simulink model "calcul_alpha_beta_gamma_v2"  (R2024b)
settings: Solver=FixedStepDiscrete  StartTime=0.0  StopTime=10.0  FixedStep=Ts  RelTol=1e-3
values from neighbouring files (symbols this model uses):
  lf = L*fr    (= 0.7905)    [main_data_vehicle.m]    (also in xopt_launch.mat)
  lr = L-lf    (= 0.7595)    [main_data_vehicle.m]    (also in xopt_launch.mat)
settings Model: Creator=marti  LastModifiedBy=marti

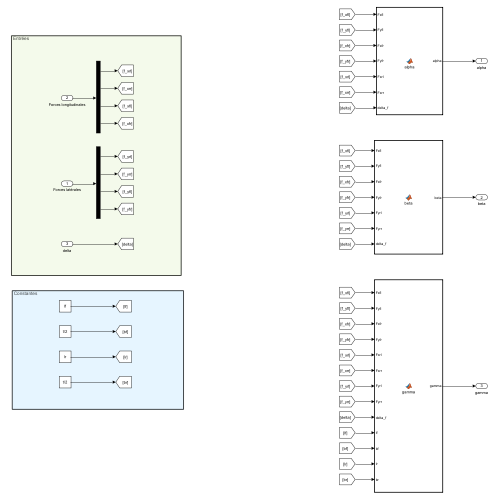
[thumbnail: Simulink's stored preview of the top-level diagram]
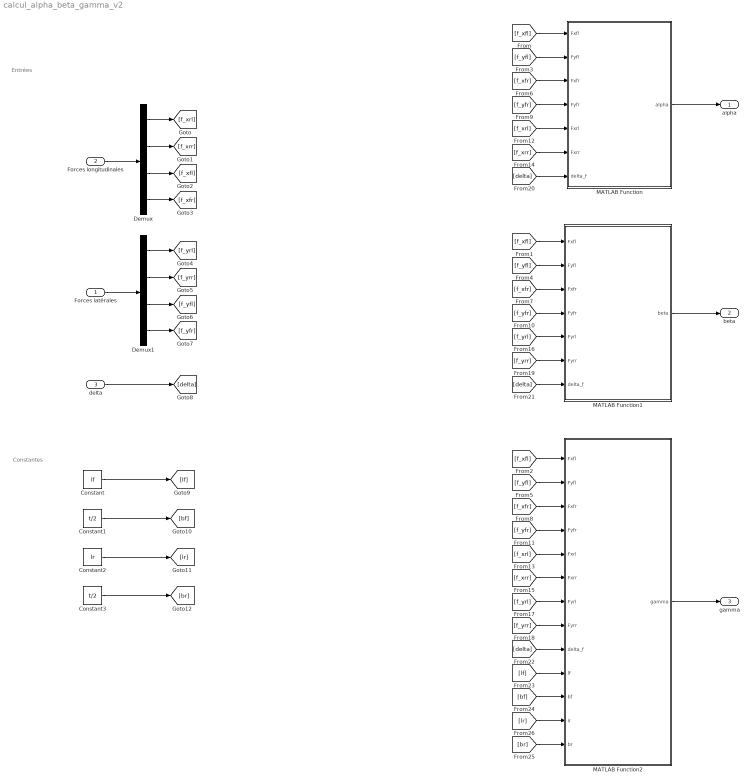
== system calcul_alpha_beta_gamma_v2 ==
  note: Constantes
  note: Entrées
  Forces latérales : Inport
  Forces longitudinales : Inport  Port=2
  delta : Inport  Port=3
  Constant : Constant  Value=lf
  Constant1 : Constant  Value=t/2
  Constant2 : Constant  Value=lr
  Constant3 : Constant  Value=t/2
  Demux : Demux
  Demux1 : Demux
  MATLAB Function : MATLAB Function  TreatAsAtomicUnit=on
  MATLAB Function1 : MATLAB Function  TreatAsAtomicUnit=on
  MATLAB Function2 : MATLAB Function  TreatAsAtomicUnit=on
  alpha : Outport
  beta : Outport  Port=2
  gamma : Outport  Port=3
  wires:
  Forces longitudinales/1 -> Demux/1
  Demux/1 -> [f_xrl]
  Demux/2 -> [f_xrr]
  Demux/3 -> [f_xfl]
  Demux/4 -> [f_xfr]
  Demux1/3 -> [f_yfl]
  Demux1/4 -> [f_yfr]
  Demux1/1 -> [f_yrl]
  Forces latérales/1 -> Demux1/1
  Demux1/2 -> [f_yrr]
  Constant/1 -> [lf]
  Constant1/1 -> [bf]
  Constant2/1 -> [lr]
  Constant3/1 -> [br]
  [f_xfl] -> MATLAB Function/1(Fxfl)
  [f_xfl] -> MATLAB Function1/1(Fxfl)
  [f_xfl] -> MATLAB Function2/1(Fxfl)
  [f_yfl] -> MATLAB Function/2(Fyfl)
  [f_yfl] -> MATLAB Function1/2(Fyfl)
  [f_yfl] -> MATLAB Function2/2(Fyfl)
  [f_xfr] -> MATLAB Function/3(Fxfr)
  [f_xfr] -> MATLAB Function1/3(Fxfr)
  [f_xfr] -> MATLAB Function2/3(Fxfr)
  [f_yfr] -> MATLAB Function/4(Fyfr)
  [f_yfr] -> MATLAB Function1/4(Fyfr)
  [f_yfr] -> MATLAB Function2/4(Fyfr)
  [f_xrl] -> MATLAB Function/5(Fxrl)
  [f_xrl] -> MATLAB Function2/5(Fxrl)
  [f_xrr] -> MATLAB Function/6(Fxrr)
  [f_xrr] -> MATLAB Function2/6(Fxrr)
  [f_yrl] -> MATLAB Function1/5(Fyrl)
  [f_yrl] -> MATLAB Function2/7(Fyrl)
  [f_yrr] -> MATLAB Function2/8(Fyrr)
  [f_yrr] -> MATLAB Function1/6(Fyrr)
  [delta] -> MATLAB Function/7(delta_f)
  [delta] -> MATLAB Function1/7(delta_f)
  [delta] -> MATLAB Function2/9(delta_f)
  [lf] -> MATLAB Function2/10(lf)
  [bf] -> MATLAB Function2/11(bf)
  [br] -> MATLAB Function2/13(br)
  [lr] -> MATLAB Function2/12(lr)
  MATLAB Function/1(alpha) -> alpha/1
  MATLAB Function1/1(beta) -> beta/1
  MATLAB Function2/1(gamma) -> gamma/1
  delta/1 -> [delta]

== matlab function calcul_alpha_beta_gamma_v2/MATLAB Function1 ==
  data: Fxfl input; beta output; Fyfl input; Fxfr input; Fyfr input; Fyrl input; Fyrr input; delta_f input
function beta = beta(Fxfl, Fyfl, Fxfr, Fyfr, Fyrl, Fyrr, delta_f)
% Calcule le terme de droite de la deuxième équation du système
% beta = Fxfl*sin(delta_f) + Fyfl*cos(delta_f) + Fxfr*sin(delta_f) + Fyfr*cos(delta_f) + Fyrl + Fyrr

beta = Fxfl*sin(delta_f) + Fyfl*cos(delta_f) + ...
       Fxfr*sin(delta_f) + Fyfr*cos(delta_f) + ...
       Fyrl + Fyrr;
end

== matlab function calcul_alpha_beta_gamma_v2/MATLAB Function ==
  data: Fxfl input; alpha output; Fyfl input; Fxfr input; Fyfr input; Fxrl input; Fxrr input; delta_f input
function alpha = alpha(Fxfl, Fyfl, Fxfr, Fyfr, Fxrl, Fxrr, delta_f)
% Calcule le terme de droite de la première équation du système
% alpha = Fxfl*cos(delta_f) - Fyfl*sin(delta_f) + Fxfr*cos(delta_f) - Fyfr*sin(delta_f) + Fxrl + Fxrr

alpha = Fxfl*cos(delta_f) - Fyfl*sin(delta_f) + ...
        Fxfr*cos(delta_f) - Fyfr*sin(delta_f) + ...
        Fxrl + Fxrr;
end

== matlab function calcul_alpha_beta_gamma_v2/MATLAB Function2 ==
  data: Fxfl input; gamma output; Fyfl input; Fxfr input; Fyfr input; Fxrl input; Fxrr input; Fyrl input; Fyrr input; delta_f input; lf input; bf input; lr input; br input
function gamma = gamma(Fxfl, Fyfl, Fxfr, Fyfr, Fxrl, Fxrr, Fyrl, Fyrr, delta_f, lf, bf, lr, br)
% Calcule le terme de droite de la troisième équation du système
% gamma = lf*(Fxfl*sin(delta_f) + Fxfr*sin(delta_f) + Fyfl*cos(delta_f) + Fyfr*cos(delta_f)) ...
%       + bf*(-Fxfl*cos(delta_f) + Fxfr*cos(delta_f) + Fyfl*sin(delta_f) - Fyfr*sin(delta_f)) ...
%       - lr*(Fyrl + Fyrr) - br*(Fxrl - Fxrr)

gamma = lf*(Fxfl*sin(delta_f) + Fxfr*sin(delta_f) + Fyfl*cos(delta_f) + Fyfr*cos(delta_f)) ...
       + bf*(-Fxfl*cos(delta_f) + Fxfr*cos(delta_f) + Fyfl*sin(delta_f) - Fyfr*sin(delta_f)) ...
       - lr*(Fyrl + Fyrr) - br*(Fxrl - Fxrr);
end
